simulink model "RandomizedBlendingCarControl"  (R2018a)
settings: Solver=VariableStepAuto  StartTime=0.0  StopTime=20  RelTol=1e-3
undefined symbols (not defined in the file): Ts, Vx
libraries: simulink x4, cstblocks x1
settings Model: Creator=The MathWorks, Inc.  LastModifiedBy=Yves
settings CodeAppCC: StateflowObjectComments=on
settings SimscapeCC: SimscapeNormalizeSystem=off

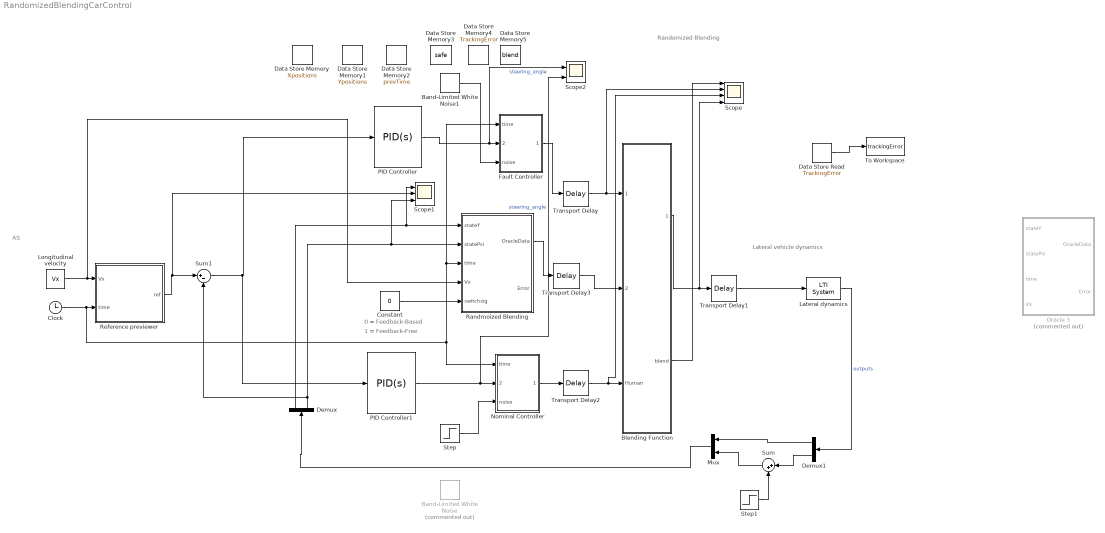
== system RandomizedBlendingCarControl ==
  note: 1 = Feedback-Free
  note: 0 = Feedback-Based
  note: Randomized Blending
  note: Lateral vehicle dynamics
  note: AS
  Band-Limited White Noise : simulink/Sources/Band-Limited White Noise  Commented=on  Cov=[0]  Ts=1  seed=[23341]
  Band-Limited White Noise1 : simulink/Sources/Band-Limited White Noise  Cov=[0]  Ts=1  seed=[23341]
  "Blending Function " : MATLAB Function  TreatAsAtomicUnit=on
  Clock : Clock
  Constant : Constant  Value=0
  Data Store Memory : DataStoreMemory  DataStoreName=Xpositions  ReadBeforeWriteMsg=warning  WriteAfterWriteMsg=warning  WriteAfterReadMsg=warning  ShowAdditionalParam=off  OutDataTypeStr=double  Dimensions=[1,5]
  Data Store Memory1 : DataStoreMemory  DataStoreName=Ypositions  ReadBeforeWriteMsg=warning  WriteAfterWriteMsg=warning  WriteAfterReadMsg=warning  ShowAdditionalParam=off  OutDataTypeStr=double  Dimensions=[1,5]
  Data Store Memory2 : DataStoreMemory  DataStoreName=prevTime  ReadBeforeWriteMsg=warning  WriteAfterWriteMsg=warning  WriteAfterReadMsg=warning  ShowAdditionalParam=off  OutDataTypeStr=double
  Data Store Memory3 : DataStoreMemory  DataStoreName=safe  ReadBeforeWriteMsg=warning  WriteAfterWriteMsg=warning  WriteAfterReadMsg=warning  ShowAdditionalParam=off  OutDataTypeStr=double
  Data Store Memory4 : DataStoreMemory  DataStoreName=TrackingError  ReadBeforeWriteMsg=warning  WriteAfterWriteMsg=warning  WriteAfterReadMsg=warning  ShowAdditionalParam=off  OutDataTypeStr=double
  Data Store Memory5 : DataStoreMemory  DataStoreName=blend  ReadBeforeWriteMsg=warning  WriteAfterWriteMsg=warning  WriteAfterReadMsg=warning  ShowAdditionalParam=off  OutDataTypeStr=double
  Data Store Read : DataStoreRead  DataStoreName=TrackingError  DataStoreElements=TrackingError
  Demux : Demux  Outputs=2
  Demux1 : Demux  Outputs=2
  Fault Controller : MATLAB Function  TreatAsAtomicUnit=on  SystemSampleTime=0.1
  Lateral dynamics : cstblocks/LTI System  sys=vehicle  IC=[]
  Longitudinal velocity : Constant  Value=Vx  SampleTime=Ts
  Mux : Mux  Inputs=2
  Nominal Controller : MATLAB Function  TreatAsAtomicUnit=on  SystemSampleTime=0.1
  Oracle 3 : MATLAB Function  Commented=on  TreatAsAtomicUnit=on  SystemSampleTime=0.1
  PID Controller : simulink/Continuous/PID Controller  Controller=PID  TimeDomain=Continuous-time  SampleTime=-1  IntegratorMethod=Forward Euler  FilterMethod=Forward Euler  Form=Parallel  UseFilter=on  ControllerParametersSource=internal  P=2  I=1  D=0.5  N=100  InitialConditionSource=internal  InitialConditionForIntegrator=0  InitialConditionForFilter=0  ExternalReset=none  LimitOutput=off  UpperSaturationLimit=inf  LowerSaturationLimit=-inf  LinearizeAsGain=on  AntiWindupMode=none  Kb=1  TrackingMode=off  Kt=1  PParamMin=[]  PParamMax=[]  IParamMin=[]  IParamMax=[]  DParamMin=[]  DParamMax=[]  NParamMin=[]  NParamMax=[]  KbParamMin=[]  KbParamMax=[]  KtParamMin=[]  KtParamMax=[]  POutMin=[]  POutMax=[]  IOutMin=[]  IOutMax=[]  DOutMin=[]  DOutMax=[]  NOutMin=[]  NOutMax=[]  KbOutMin=[]  KbOutMax=[]  KtOutMin=[]  KtOutMax=[]  IntegratorOutMin=[]  IntegratorOutMax=[]  FilterOutMin=[]  FilterOutMax=[]  SumOutMin=[]  SumOutMax=[]  SumI1OutMin=[]  SumI1OutMax=[]  SumI2OutMin=[]  SumI2OutMax=[]  SumI3OutMin=[]  SumI3OutMax=[]  SumDOutMin=[]  SumDOutMax=[]  SaturationOutMin=[]  SaturationOutMax=[]  IntegratorContinuousStateAttributes=''  IntegratorStateMustResolveToSignalObject=off  IntegratorRTWStateStorageClass=Auto  FilterContinuousStateAttributes=''  FilterStateMustResolveToSignalObject=off  FilterRTWStateStorageClass=Auto  DifferentiatorICPrevScaledInput=0  DifferentiatorOutMin=[]  DifferentiatorOutMax=[]  FilterDiffOutCoefMin=[]  FilterDiffOutCoefMax=[]  SumDenOutMin=[]  SumDenOutMax=[]  SumNumOutMin=[]  SumNumOutMax=[]  ReciprocalOutMin=[]  ReciprocalOutMax=[]  DivideOutMin=[]  DivideOutMax=[]  TunerSelectOption=Transfer Function Based (PID Tuner App)
  PID Controller1 : simulink/Continuous/PID Controller  Controller=PID  TimeDomain=Continuous-time  SampleTime=-1  IntegratorMethod=Forward Euler  FilterMethod=Forward Euler  Form=Parallel  UseFilter=on  ControllerParametersSource=internal  P=1  I=0.5  D=0.05  N=100  InitialConditionSource=internal  InitialConditionForIntegrator=0  InitialConditionForFilter=0  ExternalReset=none  LimitOutput=off  UpperSaturationLimit=inf  LowerSaturationLimit=-inf  LinearizeAsGain=on  AntiWindupMode=none  Kb=1  TrackingMode=off  Kt=1  PParamMin=[]  PParamMax=[]  IParamMin=[]  IParamMax=[]  DParamMin=[]  DParamMax=[]  NParamMin=[]  NParamMax=[]  KbParamMin=[]  KbParamMax=[]  KtParamMin=[]  KtParamMax=[]  POutMin=[]  POutMax=[]  IOutMin=[]  IOutMax=[]  DOutMin=[]  DOutMax=[]  NOutMin=[]  NOutMax=[]  KbOutMin=[]  KbOutMax=[]  KtOutMin=[]  KtOutMax=[]  IntegratorOutMin=[]  IntegratorOutMax=[]  FilterOutMin=[]  FilterOutMax=[]  SumOutMin=[]  SumOutMax=[]  SumI1OutMin=[]  SumI1OutMax=[]  SumI2OutMin=[]  SumI2OutMax=[]  SumI3OutMin=[]  SumI3OutMax=[]  SumDOutMin=[]  SumDOutMax=[]  SaturationOutMin=[]  SaturationOutMax=[]  IntegratorContinuousStateAttributes=''  IntegratorStateMustResolveToSignalObject=off  IntegratorRTWStateStorageClass=Auto  FilterContinuousStateAttributes=''  FilterStateMustResolveToSignalObject=off  FilterRTWStateStorageClass=Auto  DifferentiatorICPrevScaledInput=0  DifferentiatorOutMin=[]  DifferentiatorOutMax=[]  FilterDiffOutCoefMin=[]  FilterDiffOutCoefMax=[]  SumDenOutMin=[]  SumDenOutMax=[]  SumNumOutMin=[]  SumNumOutMax=[]  ReciprocalOutMin=[]  ReciprocalOutMax=[]  DivideOutMin=[]  DivideOutMax=[]  TunerSelectOption=Transfer Function Based (PID Tuner App)
  Randmoized Blending : MATLAB Function  TreatAsAtomicUnit=on  SystemSampleTime=0.1
  Reference previewer : MATLAB Function  TreatAsAtomicUnit=on  SystemSampleTime=Ts
  Scope : Scope  NumInputPorts=4
  Scope1 : Scope  NumInputPorts=3
  Scope2 : Scope  NumInputPorts=2
  Step : Step  Time=3.5  After=0  SampleTime=0
  Step1 : Step  Time=3.5  After=0.02  SampleTime=0
  Sum : Sum  Inputs=|++
  Sum1 : Sum  Inputs=|+-
  To Workspace : ToWorkspace  VariableName=trackingError  SaveFormat=Timeseries  SampleTime=-1
  Transport Delay{,1..3} (4 alike) : TransportDelay  DelayTime=0
  wires:
  Longitudinal velocity/1 -> Randmoized Blending/4(Vx), Reference previewer/1(Vx)
  Clock/1 -> Fault Controller/1(time), Randmoized Blending/3(time), Nominal Controller/1(time), Reference previewer/2(time)
  Reference previewer/1(ref) -> Sum1/1, Scope1/2
  Lateral dynamics/1 -> Demux1/1  "outputs"
  "Blending Function "/1(blendedOutput) -> Scope/4, Transport Delay1/1
  Randmoized Blending/1(OracleData) -> Transport Delay3/1
  Demux/2 -> Sum1/2, Scope1/3, Randmoized Blending/2(statePsi)
  Transport Delay/1 -> Scope/2, "Blending Function "/1(FaultSingal)
  Transport Delay1/1 -> Lateral dynamics/1
  Transport Delay2/1 -> Scope/3, "Blending Function "/3(Human)
  Transport Delay3/1 -> "Blending Function "/2(OracleData)
  Step/1 -> Nominal Controller/3(noise)
  Band-Limited White Noise1/1 -> Fault Controller/3(noise)
  PID Controller/1 -> Scope2/1, Fault Controller/2(original)  "steering_angle"
  Data Store Read/1 -> To Workspace/1
  PID Controller1/1 -> Scope2/2, Nominal Controller/2(original)  "steering_angle"
  Nominal Controller/1(NominalSignal) -> Transport Delay2/1
  Fault Controller/1(FaultSingal) -> Transport Delay/1
  "Blending Function "/2(blend) -> Scope/1
  Constant/1 -> Randmoized Blending/5(switchsig)
  Mux/1 -> Demux/1
  Sum1/1 -> PID Controller1/1, PID Controller/1
  Demux/1 -> Scope1/1, Randmoized Blending/1(stateY)
  Step1/1 -> Sum/2
  Demux1/1 -> Mux/1
  Demux1/2 -> Sum/1
  Sum/1 -> Mux/2

== matlab function RandomizedBlendingCarControl/Blending Function  ==
  data: FaultSingal input; blendedOutput output; OracleData input; Human input; blend output
function [blendedOutput, blend] = fcn(FaultSingal, OracleData, Human)


blend = 0;
blendedOutput = (FaultSingal*blend)+ ((1-blend)*Human);

%if(OracleData == 0)
 %   blendedOutput = 0;
%else
 %  blendedOutput = AS; 
end

== matlab function RandomizedBlendingCarControl/Reference previewer ==
  data: Vx input; time input; ref output
function ref = previewer(Vx,time)
% Get previewed reference trajectory

% Previw horizon is 10 sampling times (i.e. 10*0.1 = 1 seconds).
% Reference contains 2 signals (i.e. Y position and yaw angle).
%ref = zeros(10,2); 

[X, Z, Y] = doubleLaneChange(Vx,time + 0 * 0.5);
disp(Z);
ref = Z;
%% Previewing sequence
%for ct = 1:10
  % ref(ct,:) = doubleLaneChange(Vx,time + (ct-1)*0.1);
%end

== matlab function RandomizedBlendingCarControl/Randmoized Blending ==
  settings: updateMethod=DISCRETE
  data: stateY input; statePsi input; OracleData output; Xpositions data_store_memory; Ypositions data_store_memory; prevTime data_store_memory; time input; Vx input; safe data_store_memory; Error output; TrackingError data_store_memory; blend data_store_memory; switchsig input
function [OracleData, Error] = fcn(stateY, statePsi, time, Vx, switchsig)

obstacleX = [10,25,10,25,55,65,55,65,120,180,120,180];
obstacleY = [2,2,-1,-1,3,3,5,5,1,1,-4,-4];

global Xpositions ;
global prevTime;
global Ypositions ;
global safe; 
global TrackingError; 
global blend;

y = stateY;
psi = statePsi;

currentX = time * Vx;

collisionCourse = false;

if(prevTime+0.1 < time)
    
    prevTime = time;
    %get x and y position and add them to sliding window 
    
    Xpositions(1) = Xpositions(2);
    Xpositions(2) = Xpositions(3);
    Xpositions(3) = Xpositions(4);
    Xpositions(4) = Xpositions(5);
    Xpositions(5) = currentX;

    Ypositions(1) = Ypositions(2);
    Ypositions(2) = Ypositions(3);
    Ypositions(3) = Ypositions(4);
    Ypositions(4) = Ypositions(5);
    Ypositions(5) = y;
    
    p = polyfit(Xpositions,Ypositions,3);
    
    referencePath = zeros(3,2); 
    actualPath = zeros(3,2); 
    for ct = 1:3
       referencePath(ct,:) = doubleLaneChange(Vx,time + (ct-1)*0.1);
    end
    
    for ct2 = 1:3
       actualPath(ct2,:) = polyval(p, Vx*(time+(ct2-1)*0.1));
    end
    
    errorDif = abs(actualPath(1) - referencePath(1,1));
    isNotValid = isnan(errorDif);
    if(~isNotValid)
        %feedback-based randomized blending
        if(switchsig == 0)
            if(errorDif > 0.5)
                blend = rand;
                TrackingError = TrackingError + errorDif;
            else
                blend = 0;
            end
        else
            blend = rand;
            TrackingError = TrackingError + errorDif;
                       
        end
    end
    
     
    %check if on collision course
    %for index = 1:numel(obstacleX)
     %   obsX = obstacleX(index);
        %filter out obstacles within 5 meters
      %  if(obsX >= currentX && obsX <= currentX+5)
        %    disp('Obs in range');
         %   obsY = obstacleY(index);
         %   trajectoryForObs = polyval(p, obsX);
            
          %  disp(trajectoryForObs);
            %check if obstacle is within 0.5 meters of car
          %  if(abs(trajectoryForObs - obsY)<0.5)
           %     disp('Collosion course');
           %     collisionCourse = true;
           %    break;
           % end
      %  end
   % end
    
    
    %if(collisionCourse)
    %    blend = 0.5;
   % end
end

if(blend > 1)
    blend = 1;
end
%Safe = 0 , Unsafe = 1
OracleData = blend;
Error = TrackingError;
%disp(errorDif);

end

== matlab function RandomizedBlendingCarControl/Nominal Controller ==
  settings: updateMethod=DISCRETE
  data: time input; original input; noise input; NominalSignal output; Xpositions data_store_memory; Ypositions data_store_memory; prevTime data_store_memory; safe data_store_memory; TrackingError data_store_memory
function NominalSignal = fcn(time, original, noise)

if(time > 3 && time < 4)
    NominalSignal = original + noise;
else
    NominalSignal = original;

end

end

== matlab function RandomizedBlendingCarControl/Fault Controller ==
  settings: updateMethod=DISCRETE
  data: time input; original input; noise input; FaultSingal output; Xpositions data_store_memory; Ypositions data_store_memory; prevTime data_store_memory; safe data_store_memory; TrackingError data_store_memory
function FaultSingal = fcn(time, original, noise)

if(time > 3 && time < 4)
    FaultSingal = original + noise;
else
    FaultSingal = original;

end

end

== matlab function RandomizedBlendingCarControl/Oracle 3 ==
  settings: updateMethod=DISCRETE
  data: stateY input; statePsi input; OracleData output; Xpositions data_store_memory; Ypositions data_store_memory; prevTime data_store_memory; time input; Vx input; safe data_store_memory; Error output; TrackingError data_store_memory; blend data_store_memory
function [OracleData, Error] = fcn(stateY, statePsi, time, Vx)

obstacleX = [10,25,10,25,55,65,55,65,120,180,120,180];
obstacleY = [2,2,-1,-1,3,3,5,5,1,1,-4,-4];

global Xpositions ;
global prevTime;
global Ypositions ;
global safe; 
global TrackingError; 
global blend;

y = stateY;
psi = statePsi;

currentX = time * Vx;

collisionCourse = false;

if(prevTime+0.1 < time)
    
    prevTime = time;
    %get x and y position and add them to sliding window 
    
    Xpositions(1) = Xpositions(2);
    Xpositions(2) = Xpositions(3);
    Xpositions(3) = Xpositions(4);
    Xpositions(4) = Xpositions(5);
    Xpositions(5) = currentX;

    Ypositions(1) = Ypositions(2);
    Ypositions(2) = Ypositions(3);
    Ypositions(3) = Ypositions(4);
    Ypositions(4) = Ypositions(5);
    Ypositions(5) = y;
    
    p = polyfit(Xpositions,Ypositions,3);
    
    referencePath = zeros(3,2); 
    actualPath = zeros(3,2); 
    for ct = 1:3
       referencePath(ct,:) = doubleLaneChange(Vx,time + (ct-1)*0.1);
    end
    
    for ct2 = 1:3
       actualPath(ct2,:) = polyval(p, Vx*(time+(ct2-1)*0.1));
    end
    
    errorDif = abs(actualPath(1) - referencePath(1,1));
    isNotValid = isnan(errorDif);
    if(~isNotValid)
        blend = abs(actualPath(1) - referencePath(1,1));
        TrackingError = TrackingError + blend;
        disp(blend);
    end
    
     
    %check if on collision course
    %for index = 1:numel(obstacleX)
     %   obsX = obstacleX(index);
        %filter out obstacles within 5 meters
      %  if(obsX >= currentX && obsX <= currentX+5)
        %    disp('Obs in range');
         %   obsY = obstacleY(index);
         %   trajectoryForObs = polyval(p, obsX);
            
          %  disp(trajectoryForObs);
            %check if obstacle is within 0.5 meters of car
          %  if(abs(trajectoryForObs - obsY)<0.5)
           %     disp('Collosion course');
           %     collisionCourse = true;
           %    break;
           % end
      %  end
   % end
    
    
    %if(collisionCourse)
    %    blend = 0.5;
   % end
end

if(blend > 1)
    blend = 1;
end
%Safe = 0 , Unsafe = 1
OracleData = blend;
Error = TrackingError;
disp(TrackingError);

end
